simulink model "Arizona_base_GOAT"  (R2022a)
settings: Solver=FixedStepDiscrete  StartTime=0.0  StopTime=inf  FixedStep=Ts  RelTol=1e-3  EnableMultiTasking=on
undefined symbols (not defined in the file): DiscIntNeverNeededParam, Ended, IO307, N_Init, Nref, phi_Init, Single, x_Init, y_Init
libraries: speedgoatlib_fpga_dio x30, speedgoatlib_fpga_quadrature x19, simulink x10, speedgoatlib_IO141 x9, xpcobsoletelib x7, speedgoatlib_fpga x3, cstblocks x3
(part 1 of 3)
settings Model: SimulationMode=external  ExtModeTrigDuration=5  Creator=JBolder  LastModifiedBy=Arizona_PC
settings SolverCC: ConcurrentTasks=on  AlgebraicLoopSolver=TrustRegion  PositivePriorityOrder=on
settings DataIOCC: LimitDataPoints=on  SaveFormat=Array  ReturnWorkspaceOutputs=off  SignalLoggingName=logsOut
settings OptimizationCC: BlockReduction=off  OptimizeBlockIOStorage=off  BufferReuse=off  GlobalBufferReuse=off  ExpressionFolding=off  LocalBlockOutputs=off
settings DebuggingCC: SolverPrmCheckMsg=warning  TasksWithSamePriorityMsg=none  UnconnectedInputMsg=warning  UnconnectedOutputMsg=warning  UnconnectedLineMsg=warning  SFUnexpectedBacktrackingDiag=warning  SFNoUnconditionalDefaultTransitionDiag=warning  SFExecutionAtInitializationDiag=none  SFMachineParentedDataDiag=warning  ArithmeticOperatorsInVariantConditions=warning
settings HardwareCC: ProdBitPerLong=64  ProdLongLongMode=on  ProdHWDeviceType=Intel->x86-64 (Linux 64)
settings ModelReferenceCC: UpdateModelReferenceTargets=Force  EnableParallelModelReferenceBuilds=on  ParallelModelReferenceMATLABWorkerInit=Copy Base Workspace  PropagateVarSize=During execution  PropagateSignalLabelsOutOfModel=off
settings SFSimCC: SimUseLocalCustomCode=off  CustomCodeUndefinedFunction=UseInterfaceOnly  SimTargetLang=C++
settings RTWCC: Description=Simulink Real-Time  SystemTargetFile=slrealtime.tlc  TemplateMakefile=slrealtime_default_tmf  RTWUseLocalCustomCode=off  Toolchain=Simulink Real-Time Toolchain  BuildConfiguration=Faster Runs  CodeExecutionProfiling=on  TargetLang=C++
settings CodeAppCC: StateflowObjectComments=on
settings SimulinkRealTimeTargetCC: UseGCCFastMath=on
settings ConfigComp: CovMetricSettings=dw  CovSaveCumulativeToWorkspaceVar=on  CovSaveSingleToWorkspaceVar=on  CovExternalEMLEnable=off  CovSFcnEnable=off

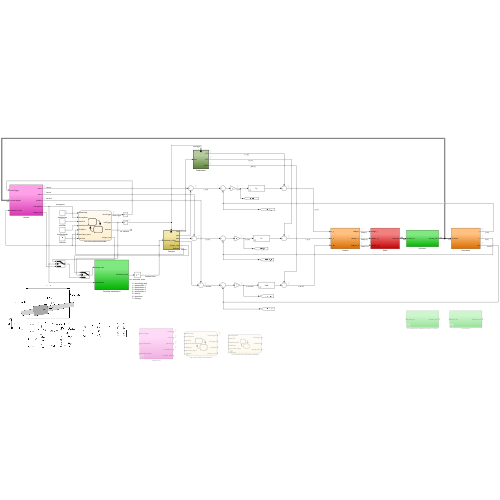
[thumbnail: Simulink's stored preview of the top-level diagram]
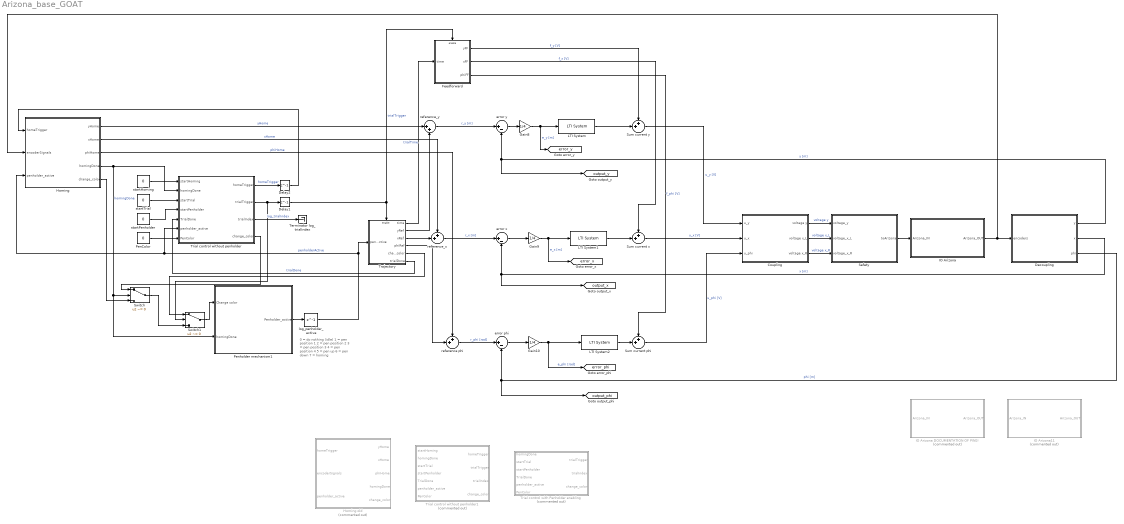
== system Arizona_base_GOAT ==
  note: 0 = do nothing (idle)
      | 1 = pen position 1
      | 2 = pen position 2
      | 3 = pen position 3
      | 4 = pen position 4
      | 5 = pen up
      | 6 = pen down
      | 7 = homing
  Coupling : Subsystem
  Decoupling : Subsystem
  Delay1 : Delay  DelayLength=1  InitialCondition=0
  Delay2 : Delay  DelayLength=1  InitialCondition=0
  Feedforward : Subsystem
  Gain10 : Gain  Gain=1/4
  Gain8 : Gain  Gain=1/4
  Gain9 : Gain  Gain=1/4
  Homing : Subsystem
  Homing old : Subsystem  Commented=on
  IO Arizona : Subsystem
  IO Arizona DOCUMENTATION OF PINS! : Subsystem  Commented=on
  IO Arizona11 : Subsystem  Commented=on
  LTI System : cstblocks/LTI System  sys=Cy  IC=[]
  LTI System1 : cstblocks/LTI System  sys=Cx  IC=[]
  LTI System2 : cstblocks/LTI System  sys=Cphi  IC=[]
  PenColor : Constant  Value=0
  Penholder mechanism1 : Subsystem
  Safety : Subsystem
  Sum current phi : Sum  Inputs=++|
  Sum current x : Sum  Inputs=++|
  Sum current y : Sum  Inputs=++|
  Switch : Switch  Criteria=u2 ~= 0  SaturateOnIntegerOverflow=off  InputSameDT=off
  Switch1 : Switch  Criteria=u2 ~= 0  SaturateOnIntegerOverflow=off  InputSameDT=off
  Terminator log_trialIndex : Terminator
  Trajectory : Subsystem  TreatAsAtomicUnit=on
  Trial control with Penholder enabling : Stateflow chart  Commented=on  TreatAsAtomicUnit=on
  Trial control without penholder : Stateflow chart  TreatAsAtomicUnit=on
  Trial control without penholder1 : Stateflow chart  Commented=on  TreatAsAtomicUnit=on
  error phi : Sum  Inputs=|+-
  error x : Sum  Inputs=|+-
  error y : Sum  Inputs=|+-
  log_penholder_active : Delay  DelayLength=1  InitialCondition=0
  reference phi : Sum  Inputs=++|
  reference_x : Sum  Inputs=++|
  reference_y : Sum  Inputs=|++
  startHoming : Constant  Value=0
  startPenholder : Constant  Value=0
  startTrial : Constant  Value=0
  tag scope: error_phi=global, error_x=global, error_y=global, output_phi=global, output_x=global, output_y=global
  wires:
  Decoupling/2(x) -> [output_x], error x/2  "x [m]"
  IO Arizona/1(Arizona_OUT) -> Homing/2(encoderSignals), Decoupling/1(encoders)
  Safety/1(toArizona) -> IO Arizona/1(Arizona_IN)
  Trajectory/4(phiRef) -> reference phi/2
  startTrial/1 -> Trial control without penholder/3(startTrial)
  Trial control without penholder/3(trialIndex) -> Terminator log_trialIndex/1  "log_trialIndex"
  Delay1/1 -> Trajectory/Enable, Feedforward/Enable  "trialTrigger"
  error y/1 -> Gain8/1
  Homing/4(homingDone) -> Penholder mechanism1/2(homingDone), Switch/2, Trial control without penholder/2(homingDone)  "homingDone"
  reference_y/1 -> error y/1  "r_y [m]"
  Feedforward/1(yFF) -> Sum current y/1  "f_y [V]"
  reference_x/1 -> error x/1  "r_x [m]"
  reference phi/1 -> error phi/1  "r_phi [rad]"
  Sum current y/1 -> Coupling/1(u_y)  "u_y [V]"
  Decoupling/1(y) -> [output_y], error y/2  "y [m]"
  Decoupling/3(phi) -> [output_phi], error phi/2  "phi [m]"
  Sum current x/1 -> Coupling/2(u_x)  "u_x [V]"
  Sum current phi/1 -> Coupling/3(u_phi)  "u_phi [V]"
  log_penholder_active/1 -> Trajectory/1(penholder_active), Homing/3(penholder_active), Trial control without penholder/6(penholder_active)  "penholderActive"
  Trajectory/1(time) -> Feedforward/1(time)  "trialTime"
  Homing/5(change_color) -> Switch/3
  Switch1/1 -> Penholder mechanism1/1(Change color)
  Switch/1 -> Switch1/3
  Trajectory/6(trialDone) -> Trial control without penholder/5(TrialDone)  "trialDone"
  Penholder mechanism1/1(Penholder_active) -> log_penholder_active/1
  Trial control without penholder/4(change_color) -> Switch/1
  Trajectory/5(change_color) -> Switch1/1
  error phi/1 -> Gain10/1
  LTI System2/1 -> Sum current phi/2
  PenColor/1 -> Trial control without penholder/7(PenColor)
  Coupling/2(voltage x_L) -> Safety/2(voltage_x_L)  "voltage x_L"
  Coupling/3(voltage x_R) -> Safety/3(voltage_x_R)  "voltage x_R"
  Trial control without penholder/2(trialTrigger) -> Switch1/2, Delay1/1
  Trial control without penholder/1(homeTrigger) -> Delay2/1  "homeTrigger"
  Delay2/1 -> Homing/1(homeTrigger)
  startHoming/1 -> Trial control without penholder/1(startHoming)
  startPenholder/1 -> Trial control without penholder/4(startPenholder)
  Homing/1(yHome) -> reference_y/1  "yHome"
  Homing/2(xHome) -> reference_x/1  "xHome"
  Homing/3(phiHome) -> reference phi/1  "phiHome"
  Coupling/1(voltage y) -> Safety/1(voltage_y)  "voltage y"
  Gain9/1 -> [error_x], LTI System1/1  "e_x [m]"
  error x/1 -> Gain9/1
  Gain8/1 -> [error_y], LTI System/1  "e_y [m]"
  Gain10/1 -> [error_phi], LTI System2/1  "e_phi [rad]"
  Trajectory/2(yRef) -> reference_y/2
  Feedforward/2(xFF) -> Sum current x/1  "f_x [V]"
  Feedforward/3(phiFF) -> Sum current phi/1  "f_phi [V]"
  Trajectory/3(xRef) -> reference_x/2
  LTI System/1 -> Sum current y/2
  LTI System1/1 -> Sum current x/2

== system Arizona_base_GOAT/Coupling ==
  u_y : Inport
  u_x : Inport  Port=2
  u_phi : Inport  Port=3
  Gain on u_phi : Gain  Gain=1/2.62
  Gain on u_x : Gain  Gain=1/2
  Sum current x_L : Sum  Inputs=|+-
  Sum current x_R : Sum  Inputs=++|
  voltage y : Outport
  voltage x_L : Outport  Port=2
  voltage x_R : Outport  Port=3
  wires:
  u_y/1 -> voltage y/1
  u_x/1 -> Gain on u_x/1
  Gain on u_phi/1 -> Sum current x_L/2, Sum current x_R/2
  Sum current x_L/1 -> voltage x_L/1
  Sum current x_R/1 -> voltage x_R/1
  u_phi/1 -> Gain on u_phi/1
  Gain on u_x/1 -> Sum current x_L/1, Sum current x_R/1

== system Arizona_base_GOAT/Decoupling ==
  encoders : Inport
  Bus Selector : BusSelector  OutputSignals=AI encoders primair.encoder carriage,AI encoders primair.encoder gantry x2,AI encoders primair.encoder gantry x1
  Gain phi : Gain  Gain=1/2.62  OutDataTypeStr=double
  Gain x : Gain  Gain=1/2  OutDataTypeStr=double
  Sum x_L + x_R : Sum  Inputs=|++
  Sum x_R - x_L : Sum  Inputs=-+|
  y : Outport
  x : Outport  Port=2
  phi : Outport  Port=3
  wires:
  encoders/1 -> Bus Selector/1
  Bus Selector/3 -> Sum x_L + x_R/2, Sum x_R - x_L/2  "<encoder gantry x1>"
  Bus Selector/2 -> Sum x_R - x_L/1, Sum x_L + x_R/1  "<encoder gantry x2>"
  Sum x_L + x_R/1 -> Gain x/1
  Sum x_R - x_L/1 -> Gain phi/1
  Gain x/1 -> x/1
  Bus Selector/1 -> y/1  "<encoder carriage>"
  Gain phi/1 -> phi/1

== system Arizona_base_GOAT/Feedforward ==
  time : Inport
  Enable : EnablePort  StatesWhenEnabling=reset
  Direct Lookup Table phiFF : LookupNDDirect  NumberOfTableDimensions=1  TableIsInput=on  Table=[4 5 ;16 19 ]
  Direct Lookup Table xFF : LookupNDDirect  NumberOfTableDimensions=1  TableIsInput=on  Table=[4 5 ;16 19 ]
  Direct Lookup Table yFF : LookupNDDirect  NumberOfTableDimensions=1  TableIsInput=on  Table=[4 5 ;16 19 ]
  set_phiFF : Constant  Value=zeros(Nref,1)
  set_xFF : Constant  Value=zeros(Nref,1)
  set_yFF : Constant  Value=zeros(Nref,1)
  yFF : Outport
  xFF : Outport  Port=2
  phiFF : Outport  Port=3
  wires:
  Direct Lookup Table phiFF/1 -> phiFF/1  "f_phi"
  Direct Lookup Table yFF/1 -> yFF/1  "f_y"
  Direct Lookup Table xFF/1 -> xFF/1  "f_x"
  set_yFF/1 -> Direct Lookup Table yFF/2
  set_xFF/1 -> Direct Lookup Table xFF/2
  time/1 -> Direct Lookup Table yFF/1, Direct Lookup Table xFF/1, Direct Lookup Table phiFF/1
  set_phiFF/1 -> Direct Lookup Table phiFF/2

== system Arizona_base_GOAT/Homing ==
  homeTrigger : Inport
  encoderSignals : Inport  Port=2
  penholder_active : Inport  Port=3
  Enabled subsystem : Subsystem
  Memory block for homing during trials : Subsystem
      settings: PortSchema="{\"entries\":[{\"content\":{\"sides\":[{\"content\":{\"connectorIds\":[\"In1\",\"In2\",\"In3\"]},\"type\":\"ConnectorPlacement.EquallySpacedRectSide\",\"uuid\":\"529cf24d-8a38-49a6-8289-3a46dbfdbf8f\"},{\"content\":{\"connectorIds\":[\"Out1\",\"Out2\",\"Out3\"],\"side\":\"RIGHT\"},\"type\":\"ConnectorPlacement.EquallySpacedRectSide\",\"uuid\":\"39565b64-7967-4644-a7cf-4ede35236997\"},{\"content\":{\"connectorIds\":[\"In4\"],\"side\":\"TOP\"},\"type\":\"ConnectorPlacement.EquallySpacedRectSide\",\"uuid\":\"fd77b9cb-a736-4f15-bdda-ed00ce93e84f\"}]},\"type\":\"ConnectorPlacement.EquallySpacedConnector\",\"uuid\":\"703cf488-7ff6-4b61-bd86-c7430d8b35d0\"}],\"packageUris\":[\"http://schema.mathworks.com/mf0/Connector/R2020b\"],\"version\":\"1.0\"}"
  yHome : Outport
  xHome : Outport  Port=2
  phiHome : Outport  Port=3
  homingDone : Outport  Port=4
  change_color : Outport  Port=5
  tag scope: homingDone=global, phiHome=global, xHome=global, yHome=global
  wires:
  encoderSignals/1 -> Enabled subsystem/1(encoderSignals)
  penholder_active/1 -> Enabled subsystem/2(penholder_active)
  homeTrigger/1 -> Enabled subsystem/Enable, Memory block for homing during trials/4(homeTrigger)
  Enabled subsystem/4(homingDone) -> homingDone/1, [homingDone]
  Memory block for homing during trials/1(yHome_memory) -> yHome/1, [yHome]
  Enabled subsystem/5(change_color) -> change_color/1
  Enabled subsystem/3(phiHome) -> Memory block for homing during trials/3(phiHome)
  Enabled subsystem/2(xHome) -> Memory block for homing during trials/2(xHome)
  Enabled subsystem/1(yHome) -> Memory block for homing during trials/1(yHome)
  Memory block for homing during trials/3(phiHome_memory) -> phiHome/1, [phiHome]
  Memory block for homing during trials/2(xHome_memory) -> xHome/1, [xHome]

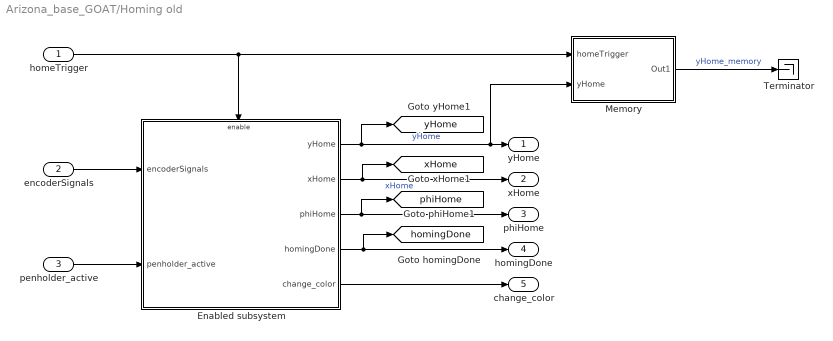
== system Arizona_base_GOAT/Homing old ==
  homeTrigger : Inport
  encoderSignals : Inport  Port=2
  penholder_active : Inport  Port=3
  Enabled subsystem : Subsystem
  Memory : Subsystem
  Terminator : Terminator
  yHome : Outport
  xHome : Outport  Port=2
  phiHome : Outport  Port=3
  homingDone : Outport  Port=4
  change_color : Outport  Port=5
  tag scope: homingDone=global, phiHome=global, xHome=global, yHome=global
  wires:
  encoderSignals/1 -> Enabled subsystem/1(encoderSignals)
  Enabled subsystem/4(homingDone) -> [homingDone], homingDone/1
  Enabled subsystem/2(xHome) -> [xHome], xHome/1  "xHome"
  Enabled subsystem/1(yHome) -> [yHome], Memory/2(yHome), yHome/1  "yHome"
  Enabled subsystem/3(phiHome) -> [phiHome], phiHome/1
  penholder_active/1 -> Enabled subsystem/2(penholder_active)
  Enabled subsystem/5(change_color) -> change_color/1
  homeTrigger/1 -> Enabled subsystem/Enable, Memory/1(homeTrigger)
  Memory/1(Out1) -> Terminator/1  "yHome_memory"

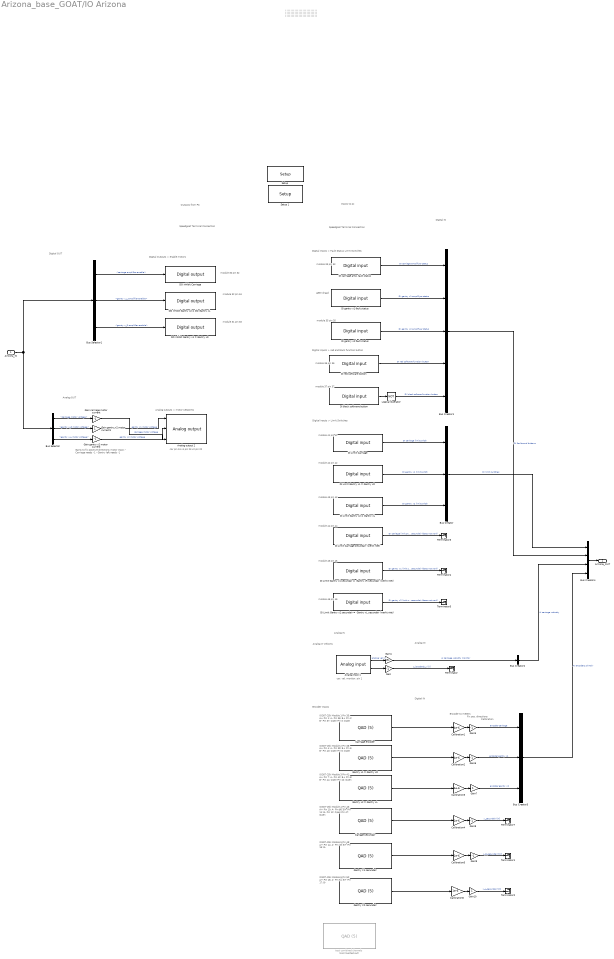
== system Arizona_base_GOAT/IO Arizona ==
  note: Inputs to pc
  note: Digital IN
  note: Speedgoat Terminal Connection
  note: Outputs from PC
  note: Speedgoat Terminal Connection
  note: Digital OUT
  note: |
      | |
      | |
      | |
      | |
      | |
      | |
      | |
      | |
      | |
      | |
      | |
      | |
      | |
      | |
      | |
      | |
      | |
      | |
      | |
      | |
      | |
      | |
      | |
      | |
      | |
      | |
      | |
      | |
      | |
      | |
      | |
      | |
      | |
      | |
      | |
      | |
      | |
      | |
      | |
      | |
      | |
      | |
      | |
      | |
      | |
      | |
      | |
      | |
      | |
      | |
      | |
      | |
      | |
      | |
      | |
      | |
      | |
      | |
      | |
      | |
      | |
      | |
      | |
      | |
      | |
      | |
      | |
      | |
      | |
      | |
      | |
  note: IO307-25k
      | Module 1
      | Pin 35: A+
      | Pin 1: A-
      | Pin 36: B+
      | Pin 2: B-
      | Pin 37: Open
      | Pin 3: Open
  note: Encoder Inputs
  note: IO307-25k
      | Module 4
      | Pin 45: A+
      | Pin 10: A-
      | Pin 46: B+
      | Pin 11: B-
      | Pin 12: Open
      | Pin 47: Open
  note: IO307-25k
      | Module 5
      | Pin 48: A+
      | Pin 14: A-
      | Pin 49: B+
      | Pin 15: B-
  note: IO307-25k
      | Module 2
      | Pin 38: A+
      | Pin 4: A-
      | Pin 39: B+
      | Pin 5: B-
      | Pin 40: Open
      | Pin 6: Open
  note: IO307-25k
      | Module 3
      | Pin 41: A+
      | Pin 7: A-
      | Pin 42: B+
      | Pin 8: B-
      | Pin 44: Open
      | Pin 10: Open
  note: IO307-25k
      | Module 6
      | Pin 50: A+
      | Pin 16: A-
      | Pin 51: B+
      | Pin 17: B-
  note: module 45
      | pin 45
  note: Digital Inputs > Limit Switches
  note: module 41
      | pin 41
  note: module 42
      | pin 42
  note: module 43
      | pin 43
  note: module 44
      | pin 44
  note: module 46
      | pin 46
  note: Digital Outputs > enable motors
  note: module 31
      | pin 33
  note: module 32
      | pin 34
  note: module 30
      | pin 32
  note: Digital inputs > red and black function button
  note: module 35
      | pin 35
  note: Digital Inputs > Fault Status Limit Switches
  note: module 36
      | pin 36
  note: module 37
      | pin 37
  note: module 33
      | pin 33
  note: geen draad
  note: Analog outputs > motor setpoints
  note: car pin 24
      | x1 pin 23
      | x2 pin 22
  note: Analog in Velocity
  note: car. vel. monitor. pin 1
  note: Analog IN
  note: Analog OUT
  note: Gains to fix positive directions motor input:
      | - Carriage needs -1
      | - Gantry left needs -1
  note: Fix pos.
      | directions
  note: Calibration
  note: Analog IN
  note: Encoder
      | to meters
  note: Digital IN
  Arizona_IN : Inport
  Analog input 1 : speedgoatlib_IO141/Analog input   parModuleId=1  parSampleTime=0.001  parPciSlot=-1  parAdcChannels=[4 9]  parAdcNumActiveChannels=[1 1]  parAdcVoltageRange=[5 5 5 5 5 5 5 5 5 5 5 5 5 5 5 5]  parAdcCoupling=[2 2]  parAdcContSampling=0  parAdcDmaEnable=0  parAdcActiveDmaDevices=[1 1 1 1]  parAdcFrameSize=100
      settings: SourceProductName=Simulink Real-Time: Speedgoat I/O Blockset
  Analog output 2 : speedgoatlib_IO141/Analog output   parModuleId=1  parSampleTime=0.001  parPciSlot=-1  parDacChannels=[2 3 4]  parDacVoltageRange=[6 6 6 6]  parDacOverRange=[1 1 1 1]  parDacInitValues=[0 0 0]  parDacReset=[1 1 1]  parDacSyncOut=0  parDacDmaEnable=0  parDacActiveDmaDevices=[1 1 1 1]  parDacDmaLatency=1  parDacFrameSize=100
      settings: SourceProductName=Simulink Real-Time: Speedgoat I/O Blockset
  Bus Creator : BusCreator  Inputs=3
  Bus Creator1 : BusCreator  Inputs=5
  Bus Creator2 : BusCreator  Inputs=1
  Bus Creator3 : BusCreator  Inputs=3
  Bus Creator4 : BusCreator  Inputs=4
  Bus Selector : BusSelector  OutputSignals=carriage motor voltage,gantry x_R motor voltage,gantry x_L motor voltage
  Bus Selector1 : BusSelector  OutputSignals=carriage amplifier enable,gantry x_L amplifier enable,gantry x_R amplifier enable
  Calibration1 : Gain  Gain=4e-6
  Calibration2 : Gain  Gain=4e-6
  Calibration3 : Gain  Gain=4e-6
  Calibration4 : Gain  Gain=1e-6
  Calibration5 : Gain  Gain=1e-6
  Calibration6 : Gain  Gain=1e-6
  Cariage secundair : speedgoatlib_fpga_quadrature/QAD (5)  id=1  chan=4  sampleTime=0.001  enableDma=on  board=IO307-25k  pciSlot=-1  numOfSlots=1  sensorType=Capture A + B Signal  interpolatePosition=on  swapAB=off  indexControlMode=Ignore Index  latchMode=Disabled  gateIndex=No Gating  speedFilterWidth=4  showInputSpeedFilterWidth=off  glitchFilterSeconds=106.7e-9  glitchFilterSecondsEff=108.5e-9  showInputClearPosition=off  showInputClearIndexFound=off  showOutputPosition=off  showOutputTurn=on  showOutputSpeed=off  showOutputIndexFound=off  showOutputLastPulse=off
      settings: SourceProductName=Simulink Real-Time: Speedgoat I/O Blockset
  Carriage encoder : speedgoatlib_fpga_quadrature/QAD (5)  id=1  chan=1  sampleTime=0.001  enableDma=on  board=IO307-25k  pciSlot=-1  numOfSlots=1  sensorType=Capture A + B Signal  interpolatePosition=on  swapAB=off  indexControlMode=Ignore Index  latchMode=Disabled  gateIndex=No Gating  speedFilterWidth=1  showInputSpeedFilterWidth=off  glitchFilterSeconds=106.7e-9  glitchFilterSecondsEff=108.5e-9  showInputClearPosition=off  showInputClearIndexFound=off  showOutputPosition=off  showOutputTurn=on  showOutputSpeed=off  showOutputIndexFound=off  showOutputLastPulse=off
      settings: SourceProductName=Simulink Real-Time: Speedgoat I/O Blockset
  "DI Limit Carriage " : speedgoatlib_fpga_dio/Digital input  id=1  chan=[41]  ts=0.001  pciSlot=-1  board=IO307-25k  vectorizeOutput=off
      settings: SourceProductName=Simulink Real-Time: Speedgoat I/O Blockset
  DI Limit Carriage secundair (werkt niet) : speedgoatlib_fpga_dio/Digital input  id=1  chan=[44]  ts=0.001  pciSlot=-1  board=IO307-25k  vectorizeOutput=off
      settings: SourceProductName=Simulink Real-Time: Speedgoat I/O Blockset
  DI Limit Gantry x1 = Gantry xR : speedgoatlib_fpga_dio/Digital input  id=1  chan=[42]  ts=0.001  pciSlot=-1  board=IO307-25k  vectorizeOutput=off
      settings: SourceProductName=Simulink Real-Time: Speedgoat I/O Blockset
  DI Limit Gantry x1 secundair =  Gantry xR secundair (werkt niet) : speedgoatlib_fpga_dio/Digital input  id=1  chan=[45]  ts=0.001  pciSlot=-1  board=IO307-25k  vectorizeOutput=off
      settings: SourceProductName=Simulink Real-Time: Speedgoat I/O Blockset
  DI Limit Gantry x2 = Gantry xL : speedgoatlib_fpga_dio/Digital input  id=1  chan=[43]  ts=0.001  pciSlot=-1  board=IO307-25k  vectorizeOutput=off
      settings: SourceProductName=Simulink Real-Time: Speedgoat I/O Blockset
  DI Limit Gantry x2 secundair =  Gantry xL secundair (werkt niet) : speedgoatlib_fpga_dio/Digital input  id=1  chan=[46]  ts=0.001  pciSlot=-1  board=IO307-25k  vectorizeOutput=off
      settings: SourceProductName=Simulink Real-Time: Speedgoat I/O Blockset
  DI black software button : speedgoatlib_fpga_dio/Digital input  id=1  chan=[37]  ts=0.001  pciSlot=-1  board=IO307-25k  vectorizeOutput=off
      settings: SourceProductName=Simulink Real-Time: Speedgoat I/O Blockset
  DI carriage amp. fault status : speedgoatlib_fpga_dio/Digital input  id=1  chan=[33]  ts=0.001  pciSlot=-1  board=IO307-25k  vectorizeOutput=off
      settings: SourceProductName=Simulink Real-Time: Speedgoat I/O Blockset
  DI gantry x1 fault status : speedgoatlib_fpga_dio/Digital input  id=1  chan=[34]  ts=0.001  pciSlot=-1  board=IO307-25k  vectorizeOutput=off
      settings: SourceProductName=Simulink Real-Time: Speedgoat I/O Blockset
  DI gantry x2 fault status : speedgoatlib_fpga_dio/Digital input  id=1  chan=[35]  ts=0.001  pciSlot=-1  board=IO307-25k  vectorizeOutput=off
      settings: SourceProductName=Simulink Real-Time: Speedgoat I/O Blockset
  DI red software button : speedgoatlib_fpga_dio/Digital input  id=1  chan=[36]  ts=0.001  pciSlot=-1  board=IO307-25k  vectorizeOutput=off
      settings: SourceProductName=Simulink Real-Time: Speedgoat I/O Blockset
  DO Inhibit Carriage : speedgoatlib_fpga_dio/Digital output  id=1  chan=[30]  init=[0]  reset=[0]  vectorizeInput=off  ts=0.001  pciSlot=-1  board=IO307-25k
      settings: SourceProductName=Simulink Real-Time: Speedgoat I/O Blockset
  DO Inhibit Gantry x1 = Gantry xR : speedgoatlib_fpga_dio/Digital output  id=1  chan=[31]  init=[0]  reset=[0]  vectorizeInput=off  ts=0.001  pciSlot=-1  board=IO307-25k
      settings: SourceProductName=Simulink Real-Time: Speedgoat I/O Blockset
  DO Inhibit Gantry x2 = DO Gantry xL : speedgoatlib_fpga_dio/Digital output  id=1  chan=[32]  init=[0]  reset=[0]  vectorizeInput=off  ts=0.001  pciSlot=-1  board=IO307-25k
      settings: SourceProductName=Simulink Real-Time: Speedgoat I/O Blockset
  Gain{,5..6,8..9} (5 alike) : Gain  Gain=-1
  Gain carriage motor current : Gain  Gain=-1
  Gain gantry x2 motor current : Gain  Gain=-1
  Gain gantry x2 motor current1 : Gain
  Gain1 : Gain  Gain=134
  Gain10 : Gain
  Gain7 : Gain
  Gantry X1 secundair : speedgoatlib_fpga_quadrature/QAD (5)  id=1  chan=5  sampleTime=0.001  enableDma=on  board=IO307-25k  pciSlot=-1  numOfSlots=1  sensorType=Capture A + B Signal  interpolatePosition=on  swapAB=off  indexControlMode=Ignore Index  latchMode=Disabled  gateIndex=No Gating  speedFilterWidth=4  showInputSpeedFilterWidth=off  glitchFilterSeconds=106.7e-9  glitchFilterSecondsEff=108.5e-9  showInputClearPosition=off  showInputClearIndexFound=off  showOutputPosition=off  showOutputTurn=on  showOutputSpeed=off  showOutputIndexFound=off  showOutputLastPulse=off
      settings: SourceProductName=Simulink Real-Time: Speedgoat I/O Blockset
  Gantry x1 = Gantry xR : speedgoatlib_fpga_quadrature/QAD (5)  id=1  chan=2  sampleTime=0.001  enableDma=on  board=IO307-25k  pciSlot=-1  numOfSlots=1  sensorType=Capture A + B Signal  interpolatePosition=on  swapAB=off  indexControlMode=Ignore Index  latchMode=Disabled  gateIndex=No Gating  speedFilterWidth=1  showInputSpeedFilterWidth=off  glitchFilterSeconds=106.7e-9  glitchFilterSecondsEff=108.5e-9  showInputClearPosition=off  showInputClearIndexFound=off  showOutputPosition=off  showOutputTurn=on  showOutputSpeed=off  showOutputIndexFound=off  showOutputLastPulse=off
      settings: SourceProductName=Simulink Real-Time: Speedgoat I/O Blockset
  Gantry x2 = Gantry xL : speedgoatlib_fpga_quadrature/QAD (5)  id=1  chan=3  sampleTime=0.001  enableDma=on  board=IO307-25k  pciSlot=-1  numOfSlots=1  sensorType=Capture A + B Signal  interpolatePosition=on  swapAB=off  indexControlMode=Ignore Index  latchMode=Disabled  gateIndex=No Gating  speedFilterWidth=1  showInputSpeedFilterWidth=off  glitchFilterSeconds=106.7e-9  glitchFilterSecondsEff=108.5e-9  showInputClearPosition=off  showInputClearIndexFound=off  showOutputPosition=off  showOutputTurn=on  showOutputSpeed=off  showOutputIndexFound=off  showOutputLastPulse=off
      settings: SourceProductName=Simulink Real-Time: Speedgoat I/O Blockset
  Gentry X2 secundair : speedgoatlib_fpga_quadrature/QAD (5)  id=1  chan=6  sampleTime=0.001  enableDma=on  board=IO307-25k  pciSlot=-1  numOfSlots=1  sensorType=Capture A + B Signal  interpolatePosition=on  swapAB=off  indexControlMode=Ignore Index  latchMode=Disabled  gateIndex=No Gating  speedFilterWidth=4  showInputSpeedFilterWidth=off  glitchFilterSeconds=106.7e-9  glitchFilterSecondsEff=108.5e-9  showInputClearPosition=off  showInputClearIndexFound=off  showOutputPosition=off  showOutputTurn=on  showOutputSpeed=off  showOutputIndexFound=off  showOutputLastPulse=off
      settings: SourceProductName=Simulink Real-Time: Speedgoat I/O Blockset
  Logical Operator : Logic  Operator=NOT  AllPortsSameDT=off  OutDataTypeStr=boolean
  Setup : speedgoatlib_fpga/Setup/Setup  board=IO307-25k  id=1  device_id=1  frontIO=None  rearIO=None  bitstreamFile=speedgoat_IO307_25k_CI_02479  rev=1.000000  timestamp_string=28/12/21 17:14:03  fpgaFreq=73.73 MHz  fpgaTick=13.56 ns  ProgSpiFlash=off  ProgBPIFlash=off  pciSlot=-1  PullRPort0=pull-up 3.3V  VioPort0=3.3V  PullRPort1=pull-up 3.3V  VioPort1=3.3V  PullRPort2=pull-up 3.3V  VioPort2=3.3V  PullRPort3=pull-up 3.3V  VioPort3=3.3V  PullRPort4=pull-up 3.3V  VioPort4=3.3V  PullRPort5=pull-up 3.3V  VioPort5=3.3V  PullRPort6=pull-up 3.3V  VioPort6=3.3V  PullRPort15=pull-up 3.3V  PullRPort31=pull-up 3.3V  PullRPort47=pull-up 3.3V  PullRPort63=pull-up 3.3V  diffLineTermination_1=on  diffLineTermination_2=on  diffLineTermination_3=on  diffLineTermination_4=on  diffLineTermination_5=on  diffLineTermination_6=on  diffLineTermination_7=on  diffLineTermination_8=on
      settings: SourceProductName=Simulink Real-Time: Speedgoat I/O Blockset
  Setup 1 : speedgoatlib_IO141/Setup   parPciSlot=-1  parModuleId=1  parInterModuleSync=Independent  parConvClockBaseRate=20MHz  parConvClock1Divider=20000  parConvClock2Divider=20000  parFrameTriggerEnable=off  parFrameTriggerDivider=10  parConvClock1BaseRate=1  parConvClock2BaseRate=1  parFrameTriggerClock=1  parAdcCoupling1=Single-Ended  parAdcChannels1=[1 2]  parAdcChannel11=off  parAdcChannel12=off  parAdcChannel13=off  parAdcChannel14=on  parAdcChannel15=off  parAdcChannel16=off  parAdcChannel17=off  parAdcChannel18=off  parAdcRangeAll1=+-10.24 V  parVoltageRangePerChannelEn1=off  parAdcRange11=+-0.64 V  parAdcRange12=+-0.64 V  parAdcRange13=+-0.64 V  parAdcRange14=+-0.64 V  parAdcRange15=+-0.64 V  parAdcRange16=+-0.64 V  parAdcRange17=+-0.64 V  parAdcRange18=+-0.64 V  parAdcCoupling2=Single-Ended  parAdcChannels2=[9 10]  parAdcChannel21=on  parAdcChannel22=off  parAdcChannel23=off  parAdcChannel24=off  parAdcChannel25=off  parAdcChannel26=off  parAdcChannel27=off  parAdcChannel28=off  parAdcRangeAll2=+-10.24 V  parVoltageRangePerChannelEn2=off  parAdcRange21=+-0.64 V  parAdcRange22=+-0.64 V  parAdcRange23=+-0.64 V  parAdcRange24=+-0.64 V  parAdcRange25=+-0.64 V  parAdcRange26=+-0.64 V  parAdcRange27=+-0.64 V  parAdcRange28=+-0.64 V  parAdcChannels=[4 9]  parAdcNumActiveChannels=[1 1]  parAdcVoltageRange=[5 5 5 5 5 5 5 5 5 5 5 5 5 5 5 5]  parAdcCoupling=[2 2]  parAdcContSampling=off  parAdcAutoCorrection=on  parAdcDmaEnable=off  parAdcDmaClock=Clock 1  parAdcFrameSize_=100  parAdcSampleTime_=-1  parAdcActiveDmaDevices=[1 1 1 1]  parAdcFrameTriggerEnable=0  parAdcFrameSize=100  parAdcSampleTime=0.1  parDacChannels=[1 2]  parDacChannel1=off  parDacChannel2=on  parDacChannel3=on  parDacChannel4=on  parDacInitValues=0  parDacResets=1  parDacVoltageRange=[6 6 6 6]  parDacOverRange=[1 1 1 1]  parDacRange1=+-6 V  parDacInitValue1=0  parDacReset1=on  parDacRange2=+-6 V  parDacInitValue2=0  parDacReset2=on  parDacRange3=+-6 V  parDacInitValue3=0  parDacReset3=on  parDacRange4=+-6 V  parDacInitValue4=0  parDacReset4=on  parDacAutoCorrection=on  parDacSyncOut=off  parDacDmaEnable=off  parDacDmaLatency=As small as possible  parDacDmaClock=Clock 1  parDacFrameSize_=100  parDacSampleTime_=-1  parDacActiveDmaDevices=[1 1 1 1]  parDacFrameTriggerEnable=0  parDacFrameSize=100  parDacSampleTime=0.1  parDiChannels=[1 2 3 4 5]  parDoChannels=[6 7 8]  parDioChannel1=In  parDioChannel2=In  parDioChannel3=In  parDioChannel4=In  parDioChannel5=In  parDioChannel6=Out  parDioChannel7=Out  parDioChannel8=Out  parDoInitValues=[0 1 0]  parDoReset=[1 1 1]  parDoInitValue1=0  parDoReset1=on  parDoInitValue2=0  parDoReset2=on  parDoInitValue3=0  parDoReset3=on  parDoInitValue4=0  parDoReset4=on  parDoInitValue5=0  parDoReset5=on  parDoInitValue6=0  parDoReset6=on  parDoInitValue7=1  parDoReset7=on  parDoInitValue8=0  parDoReset8=on  parDiDebounceEnable=off  parDiDebounceTime=0  parDiDebounceValue=0  parDioPullRefFront=Pull-up 3.3 V  parDioPullRefRear=Floating
      settings: SourceProductName=Simulink Real-Time: Speedgoat I/O Blockset
  Terminator{,1..5,7} (7 alike) : Terminator
  test combined channels : speedgoatlib_fpga_quadrature/QAD (5)  Commented=on  id=1  chan=[1:6]  sampleTime=0.001  enableDma=on  board=IO307-25k  pciSlot=-1  numOfSlots=[ones(1,6)]  sensorType=Capture A + B Signal  interpolatePosition=off  swapAB=off  indexControlMode=Ignore Index  latchMode=Disabled  gateIndex=No Gating  speedFilterWidth=4  showInputSpeedFilterWidth=off  glitchFilterSeconds=106.7e-9  glitchFilterSecondsEff=108.5e-9  showInputClearPosition=off  showInputClearIndexFound=off  showOutputPosition=off  showOutputTurn=on  showOutputSpeed=off  showOutputIndexFound=off  showOutputLastPulse=off
      settings: SourceProductName=Simulink Real-Time: Speedgoat I/O Blockset
  Arizona_OUT : Outport
  wires:
  DI black software button/1 -> Logical Operator/1
  Bus Selector1/2 -> DO Inhibit Gantry x2 = DO Gantry xL/1  "<gantry x_L amplifier enable>"
  Gain carriage motor current/1 -> Analog output 2/3  "carriage motor voltage"
  Bus Selector/2 -> Gain gantry x2 motor current1/1  "<gantry x_R motor voltage>"
  Bus Selector1/3 -> DO Inhibit Gantry x1 = Gantry xR/1  "<gantry x_R amplifier enable>"
  Gain gantry x2 motor current1/1 -> Analog output 2/1  "gantry x1 motor voltage"
  Bus Selector/1 -> Gain carriage motor current/1  "<carriage motor voltage>"
  Bus Selector1/1 -> DO Inhibit Carriage/1  "<carriage amplifier enable>"
  Arizona_IN/1 -> Bus Selector1/1, Bus Selector/1
  Gain gantry x2 motor current/1 -> Analog output 2/2  "gantry x2 motor voltage"
  Bus Selector/3 -> Gain gantry x2 motor current/1  "<gantry x_L motor voltage>"
  Gentry X2 secundair/1 -> Calibration6/1
  DI gantry x1 fault status/1 -> Bus Creator1/2  "DI gantry x1 amplifyer status"
  Cariage secundair/1 -> Calibration4/1
  Gain9/1 -> Terminator1/1  "x_R_secundair [m]"
  DI gantry x2 fault status/1 -> Bus Creator1/3  "DI gantry x2 amplifyer status"
  Gain7/1 -> Bus Creator3/3  "encoder gantry x2"
  DI Limit Gantry x2 secundair =  Gantry xL secundair (werkt niet)/1 -> Terminator5/1  "DI gantry x2 limit switch secundair (does not work)"
  Calibration2/1 -> Gain6/1
  Analog input 1/1 -> Gain1/1  "analog vel in"
  Calibration4/1 -> Gain8/1
  Gain5/1 -> Bus Creator3/1  "encoder carriage"
  DI Limit Carriage secundair (werkt niet)/1 -> Terminator3/1  "DI carriage limit switch secundair (does not work)"
  DI Limit Gantry x1 secundair =  Gantry xR secundair (werkt niet)/1 -> Terminator4/1  "DI gantry x1 limit switch secundair (does not work)"
  Gantry X1 secundair/1 -> Calibration5/1
  Gantry x1 = Gantry xR/1 -> Calibration2/1
  Gain6/1 -> Bus Creator3/2  "encoder gantry x1"
  Gantry x2 = Gantry xL/1 -> Calibration3/1
  Carriage encoder/1 -> Calibration1/1
  Bus Creator1/1 -> Bus Creator4/2  "DI faults and buttons"
  Calibration1/1 -> Gain5/1
  Bus Creator4/1 -> Arizona_OUT/1
  DI red software button/1 -> Bus Creator1/4  "DI red software function button"
  Logical Operator/1 -> Bus Creator1/5  "DI black sofware function button"
  Calibration3/1 -> Gain7/1
  Gain1/1 -> Bus Creator2/1  "AI carriage velocity monitor"
  Calibration5/1 -> Gain9/1
  Bus Creator3/1 -> Bus Creator4/4  "AI encoders primair"
  Bus Creator2/1 -> Bus Creator4/3  "AI carriage velocity"
  Gain8/1 -> Terminator7/1  "y_secundair [m]"
  DI Limit Gantry x2 = Gantry xL/1 -> Bus Creator/3  "DI gantry x2 limit switch"
  Gain10/1 -> Terminator2/1  "x_L_secundair [m]"
  DI Limit Gantry x1 = Gantry xR/1 -> Bus Creator/2  "DI gantry x1 limit switch"
  "DI Limit Carriage "/1 -> Bus Creator/1  "DI carriage limit switch"
  DI carriage amp. fault status/1 -> Bus Creator1/1  "DI carriage amplifyer status"
  Bus Creator/1 -> Bus Creator4/1  "DI limit switches"
  Calibration6/1 -> Gain10/1
  Analog input 1/2 -> Gain/1
  Gain/1 -> Terminator/1  "u_loopback_y [V]"

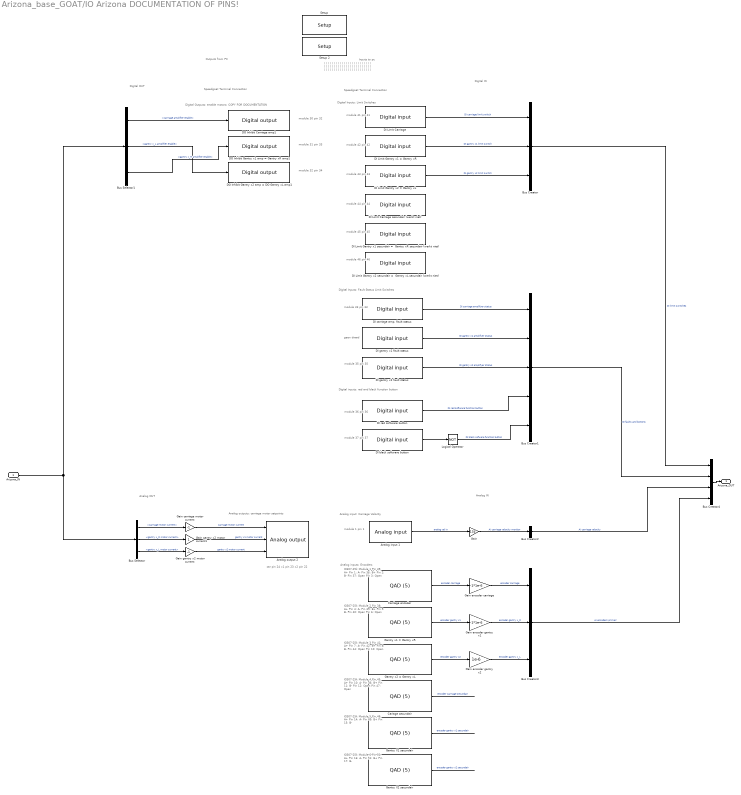
== system Arizona_base_GOAT/IO Arizona DOCUMENTATION OF PINS! ==
  note: Inputs to pc
  note: Analog IN
  note: Digital IN
  note: Speedgoat Terminal Connection
  note: Outputs from PC
  note: Speedgoat Terminal Connection
  note: IO307-25k
      | Module 6
      | Pin 50: A+
      | Pin 16: A-
      | Pin 51: B+
      | Pin 17: B-
  note: IO307-25k
      | Module 1
      | Pin 35: A+
      | Pin 1: A-
      | Pin 36: B+
      | Pin 2: B-
      | Pin 37: Open
      | Pin 3: Open
  note: IO307-25k
      | Module 5
      | Pin 48: A+
      | Pin 14: A-
      | Pin 49: B+
      | Pin 15: B-
  note: IO307-25k
      | Module 2
      | Pin 38: A+
      | Pin 4: A-
      | Pin 39: B+
      | Pin 5: B-
      | Pin 40: Open
      | Pin 6: Open
  note: Analog inputs: Encoders
  note: IO307-25k
      | Module 3
      | Pin 41: A+
      | Pin 7: A-
      | Pin 42: B+
      | Pin 8: B-
      | Pin 44: Open
      | Pin 10: Open
  note: IO307-25k
      | Module 4
      | Pin 45: A+
      | Pin 10: A-
      | Pin 46: B+
      | Pin 11: B-
      | Pin 12: Open
      | Pin 47: Open
  note: Digital Inputs: Limit Switches
  note: module 42
      | pin 42
  note: module 43
      | pin 43
  note: module 41
      | pin 41
  note: module 44
      | pin 44
  note: module 45
      | pin 45
  note: module 46
      | pin 46
  note: Digital Inputs: Fault Status Limit Switches
  note: Digital inputs: red and black function button
  note: module 37
      | pin 37
  note: geen draad
  note: module 33
      | pin 33
  note: module 35
      | pin 35
  note: module 36
      | pin 36
  note: Analog input: Carriage Velocity
  note: module 1
      | pin 1
  note: Digital OUT
  note: Analog OUT
  note: Analog outputs: carriage motor setpoints
  note: car pin 24
      | x1 pin 23
      | x2 pin 22
  note: |
      | |
      | |
      | |
      | |
      | |
      | |
      | |
      | |
      | |
      | |
      | |
      | |
      | |
      | |
      | |
      | |
      | |
      | |
      | |
      | |
      | |
      | |
      | |
      | |
      | |
      | |
      | |
      | |
      | |
      | |
      | |
      | |
      | |
      | |
      | |
      | |
      | |
      | |
      | |
      | |
      | |
      | |
      | |
      | |
      | |
      | |
      | |
      | |
      | |
      | |
      | |
      | |
      | |
      | |
      | |
      | |
      | |
      | |
      | |
      | |
      | |
      | |
      | |
      | |
      | |
      | |
      | |
      | |
      | |
      | |
      | |
  note: Digital Outputs: enable motors: COPY FOR DOCUMENTATION
  note: module 32
      | pin 34
  note: module 31
      | pin 33
  note: module 30
      | pin 32
  Arizona_IN : Inport
  Analog input 1 : speedgoatlib_IO141/Analog input   parModuleId=1  parSampleTime=0.001  parPciSlot=-1  parAdcChannels=4  parAdcNumActiveChannels=[1 0]  parAdcVoltageRange=[5 5 5 5 5 5 5 5 5 5 5 5 5 5 5 5]  parAdcCoupling=[2 1]  parAdcContSampling=0  parAdcDmaEnable=0  parAdcActiveDmaDevices=[1 1 1 1]  parAdcFrameSize=100
      settings: SourceProductName=Simulink Real-Time: Speedgoat I/O Blockset
  Analog output 2 : speedgoatlib_IO141/Analog output   parModuleId=1  parSampleTime=0.001  parPciSlot=-1  parDacChannels=[1 2 3]  parDacVoltageRange=[5 5 5 7]  parDacOverRange=[0 0 0 0]  parDacInitValues=[0 0 0]  parDacReset=[1 1 1]  parDacSyncOut=1  parDacDmaEnable=0  parDacActiveDmaDevices=[1 1 1 1]  parDacDmaLatency=1  parDacFrameSize=100
      settings: SourceProductName=Simulink Real-Time: Speedgoat I/O Blockset
  Bus Creator : BusCreator  Inputs=3
  Bus Creator1 : BusCreator  Inputs=5
  Bus Creator2 : BusCreator  Inputs=1
  Bus Creator3 : BusCreator  Inputs=3
  Bus Creator4 : BusCreator  Inputs=4
  Bus Selector : BusSelector  OutputSignals=carriage motor current,gantry x_R motor current,gantry x_L motor current
  Bus Selector1 : BusSelector  OutputSignals=carriage amplifier enable,gantry x_L amplifier enable,gantry x_R amplifier enable
  Cariage secundair : speedgoatlib_fpga_quadrature/QAD (5)  id=1  chan=[4]  sampleTime=0.001  enableDma=on  board=IO307-25k  pciSlot=-1  numOfSlots=[1]  sensorType=Capture A + B Signal  interpolatePosition=off  swapAB=off  indexControlMode=Ignore Index  latchMode=Disabled  gateIndex=No Gating  speedFilterWidth=4  showInputSpeedFilterWidth=off  glitchFilterSeconds=106.7e-9  glitchFilterSecondsEff=108.5e-9  showInputClearPosition=off  showInputClearIndexFound=off  showOutputPosition=off  showOutputTurn=on  showOutputSpeed=off  showOutputIndexFound=off  showOutputLastPulse=off
      settings: SourceProductName=Simulink Real-Time: Speedgoat I/O Blockset
  Carriage encoder : speedgoatlib_fpga_quadrature/QAD (5)  id=1  chan=[1]  sampleTime=0.001  enableDma=on  board=IO307-25k  pciSlot=-1  numOfSlots=[1]  sensorType=Capture A + B Signal  interpolatePosition=off  swapAB=off  indexControlMode=Ignore Index  latchMode=Disabled  gateIndex=No Gating  speedFilterWidth=4  showInputSpeedFilterWidth=off  glitchFilterSeconds=106.7e-9  glitchFilterSecondsEff=108.5e-9  showInputClearPosition=off  showInputClearIndexFound=off  showOutputPosition=off  showOutputTurn=on  showOutputSpeed=off  showOutputIndexFound=off  showOutputLastPulse=off
      settings: SourceProductName=Simulink Real-Time: Speedgoat I/O Blockset
  "DI Limit Carriage " : speedgoatlib_fpga_dio/Digital input  id=1  chan=[41]  ts=0.001  pciSlot=-1  board=IO307-25k  vectorizeOutput=off
      settings: SourceProductName=Simulink Real-Time: Speedgoat I/O Blockset
  DI Limit Carriage secundair (werkt niet) : speedgoatlib_fpga_dio/Digital input  id=1  chan=[44]  ts=0.001  pciSlot=-1  board=IO307-25k  vectorizeOutput=off
      settings: SourceProductName=Simulink Real-Time: Speedgoat I/O Blockset
  DI Limit Gantry x1 = Gantry xR : speedgoatlib_fpga_dio/Digital input  id=1  chan=[42]  ts=0.001  pciSlot=-1  board=IO307-25k  vectorizeOutput=off
      settings: SourceProductName=Simulink Real-Time: Speedgoat I/O Blockset
  DI Limit Gantry x1 secundair =  Gantry xR secundair (werkt niet) : speedgoatlib_fpga_dio/Digital input  id=1  chan=[45]  ts=0.001  pciSlot=-1  board=IO307-25k  vectorizeOutput=off
      settings: SourceProductName=Simulink Real-Time: Speedgoat I/O Blockset
  DI Limit Gantry x2 = Gantry xL : speedgoatlib_fpga_dio/Digital input  id=1  chan=[43]  ts=0.001  pciSlot=-1  board=IO307-25k  vectorizeOutput=off
      settings: SourceProductName=Simulink Real-Time: Speedgoat I/O Blockset
  DI Limit Gantry x2 secundair =  Gantry xL secundair (werkt niet) : speedgoatlib_fpga_dio/Digital input  id=1  chan=[46]  ts=0.001  pciSlot=-1  board=IO307-25k  vectorizeOutput=off
      settings: SourceProductName=Simulink Real-Time: Speedgoat I/O Blockset
  DI black software button : speedgoatlib_fpga_dio/Digital input  id=1  chan=[37]  ts=0.001  pciSlot=-1  board=IO307-25k  vectorizeOutput=off
      settings: SourceProductName=Simulink Real-Time: Speedgoat I/O Blockset
  DI carriage amp. fault status : speedgoatlib_fpga_dio/Digital input  id=1  chan=[33]  ts=0.001  pciSlot=-1  board=IO307-25k  vectorizeOutput=off
      settings: SourceProductName=Simulink Real-Time: Speedgoat I/O Blockset
  DI gantry x1 fault status : speedgoatlib_fpga_dio/Digital input  id=1  chan=[34]  ts=0.001  pciSlot=-1  board=IO307-25k  vectorizeOutput=off
      settings: SourceProductName=Simulink Real-Time: Speedgoat I/O Blockset
  DI gantry x2 fault status : speedgoatlib_fpga_dio/Digital input  id=1  chan=[35]  ts=0.001  pciSlot=-1  board=IO307-25k  vectorizeOutput=off
      settings: SourceProductName=Simulink Real-Time: Speedgoat I/O Blockset
  DI red software button : speedgoatlib_fpga_dio/Digital input  id=1  chan=[36]  ts=0.001  pciSlot=-1  board=IO307-25k  vectorizeOutput=off
      settings: SourceProductName=Simulink Real-Time: Speedgoat I/O Blockset
  DO Inhibit Carriage amp1 : speedgoatlib_fpga_dio/Digital output  id=1  chan=[30]  init=[0]  reset=[0]  vectorizeInput=off  ts=0.001  pciSlot=-1  board=IO307-25k
      settings: SourceProductName=Simulink Real-Time: Speedgoat I/O Blockset
  DO Inhibit Gantry x1 amp = Gantry xR amp1 : speedgoatlib_fpga_dio/Digital output  id=1  chan=[31]  init=[0]  reset=[0]  vectorizeInput=off  ts=0.001  pciSlot=-1  board=IO307-25k
      settings: SourceProductName=Simulink Real-Time: Speedgoat I/O Blockset
  DO Inhibit Gantry x2 amp = DO Gantry xL amp1 : speedgoatlib_fpga_dio/Digital output  id=1  chan=[32]  init=[0]  reset=[0]  vectorizeInput=off  ts=0.001  pciSlot=-1  board=IO307-25k
      settings: SourceProductName=Simulink Real-Time: Speedgoat I/O Blockset
  Gain : Gain  Gain=134
  Gain carriage motor current : Gain  Gain=-1
  Gain encoder carriage : Gain  Gain=-1*1e-6
  Gain encoder gantry x1 : Gain  Gain=-1*1e-6
  Gain encoder gantry x2 : Gain  Gain=1e-6
  Gain gantry x2 motor current : Gain  Gain=-1
  Gain gantry x2 motor current1 : Gain
  Gantry X1 secundair : speedgoatlib_fpga_quadrature/QAD (5)  id=1  chan=[5]  sampleTime=0.001  enableDma=on  board=IO307-25k  pciSlot=-1  numOfSlots=[1]  sensorType=Capture A + B Signal  interpolatePosition=off  swapAB=off  indexControlMode=Ignore Index  latchMode=Disabled  gateIndex=No Gating  speedFilterWidth=4  showInputSpeedFilterWidth=off  glitchFilterSeconds=106.7e-9  glitchFilterSecondsEff=108.5e-9  showInputClearPosition=off  showInputClearIndexFound=off  showOutputPosition=off  showOutputTurn=on  showOutputSpeed=off  showOutputIndexFound=off  showOutputLastPulse=off
      settings: SourceProductName=Simulink Real-Time: Speedgoat I/O Blockset
  Gantry x1 = Gantry xR : speedgoatlib_fpga_quadrature/QAD (5)  id=1  chan=[2]  sampleTime=0.001  enableDma=on  board=IO307-25k  pciSlot=-1  numOfSlots=[1]  sensorType=Capture A + B Signal  interpolatePosition=off  swapAB=off  indexControlMode=Ignore Index  latchMode=Disabled  gateIndex=No Gating  speedFilterWidth=4  showInputSpeedFilterWidth=off  glitchFilterSeconds=106.7e-9  glitchFilterSecondsEff=108.5e-9  showInputClearPosition=off  showInputClearIndexFound=off  showOutputPosition=off  showOutputTurn=on  showOutputSpeed=off  showOutputIndexFound=off  showOutputLastPulse=off
      settings: SourceProductName=Simulink Real-Time: Speedgoat I/O Blockset
  Gantry x2 = Gantry xL : speedgoatlib_fpga_quadrature/QAD (5)  id=1  chan=[3]  sampleTime=0.001  enableDma=on  board=IO307-25k  pciSlot=-1  numOfSlots=[1]  sensorType=Capture A + B Signal  interpolatePosition=off  swapAB=off  indexControlMode=Ignore Index  latchMode=Disabled  gateIndex=No Gating  speedFilterWidth=4  showInputSpeedFilterWidth=off  glitchFilterSeconds=106.7e-9  glitchFilterSecondsEff=108.5e-9  showInputClearPosition=off  showInputClearIndexFound=off  showOutputPosition=off  showOutputTurn=on  showOutputSpeed=off  showOutputIndexFound=off  showOutputLastPulse=off
      settings: SourceProductName=Simulink Real-Time: Speedgoat I/O Blockset
  Gentry X2 secundair : speedgoatlib_fpga_quadrature/QAD (5)  id=1  chan=[6]  sampleTime=0.001  enableDma=on  board=IO307-25k  pciSlot=-1  numOfSlots=[1]  sensorType=Capture A + B Signal  interpolatePosition=off  swapAB=off  indexControlMode=Ignore Index  latchMode=Disabled  gateIndex=No Gating  speedFilterWidth=4  showInputSpeedFilterWidth=off  glitchFilterSeconds=106.7e-9  glitchFilterSecondsEff=108.5e-9  showInputClearPosition=off  showInputClearIndexFound=off  showOutputPosition=off  showOutputTurn=on  showOutputSpeed=off  showOutputIndexFound=off  showOutputLastPulse=off
      settings: SourceProductName=Simulink Real-Time: Speedgoat I/O Blockset
  Logical Operator : Logic  Operator=NOT  AllPortsSameDT=off  OutDataTypeStr=boolean
  Setup : speedgoatlib_fpga/Setup/Setup  board=IO307-25k  id=1  device_id=1  frontIO=None  rearIO=None  bitstreamFile=speedgoat_IO307_25k_CI_02479  rev=1.000000  timestamp_string=28/12/21 17:14:03  fpgaFreq=73.73 MHz  fpgaTick=13.56 ns  ProgSpiFlash=off  ProgBPIFlash=off  pciSlot=-1  PullRPort0=pull-up 3.3V  VioPort0=3.3V  PullRPort1=pull-up 3.3V  VioPort1=3.3V  PullRPort2=pull-up 3.3V  VioPort2=3.3V  PullRPort3=pull-up 3.3V  VioPort3=3.3V  PullRPort4=pull-up 3.3V  VioPort4=3.3V  PullRPort5=pull-up 3.3V  VioPort5=3.3V  PullRPort6=pull-up 3.3V  VioPort6=3.3V  PullRPort15=pull-up 3.3V  PullRPort31=pull-up 3.3V  PullRPort47=pull-up 3.3V  PullRPort63=pull-up 3.3V  diffLineTermination_1=on  diffLineTermination_2=on  diffLineTermination_3=on  diffLineTermination_4=on  diffLineTermination_5=on  diffLineTermination_6=on  diffLineTermination_7=on  diffLineTermination_8=on
      settings: SourceProductName=Simulink Real-Time: Speedgoat I/O Blockset
  Setup 2 : speedgoatlib_IO141/Setup   parPciSlot=-1  parModuleId=1  parInterModuleSync=Independent  parConvClockBaseRate=20MHz  parConvClock1Divider=20000  parConvClock2Divider=20000  parFrameTriggerEnable=off  parFrameTriggerDivider=10  parConvClock1BaseRate=1  parConvClock2BaseRate=1  parFrameTriggerClock=1  parAdcCoupling1=Single-Ended  parAdcChannels1=[1 2]  parAdcChannel11=off  parAdcChannel12=off  parAdcChannel13=off  parAdcChannel14=on  parAdcChannel15=off  parAdcChannel16=off  parAdcChannel17=off  parAdcChannel18=off  parAdcRangeAll1=+-10.24 V  parVoltageRangePerChannelEn1=off  parAdcRange11=+-0.64 V  parAdcRange12=+-0.64 V  parAdcRange13=+-0.64 V  parAdcRange14=+-0.64 V  parAdcRange15=+-0.64 V  parAdcRange16=+-0.64 V  parAdcRange17=+-0.64 V  parAdcRange18=+-0.64 V  parAdcCoupling2=Differential  parAdcChannels2=[9 10]  parAdcChannel21=off  parAdcChannel22=off  parAdcChannel23=off  parAdcChannel24=off  parAdcChannel25=off  parAdcChannel26=off  parAdcChannel27=off  parAdcChannel28=off  parAdcRangeAll2=+-10.24 V  parVoltageRangePerChannelEn2=off  parAdcRange21=+-0.64 V  parAdcRange22=+-0.64 V  parAdcRange23=+-0.64 V  parAdcRange24=+-0.64 V  parAdcRange25=+-0.64 V  parAdcRange26=+-0.64 V  parAdcRange27=+-0.64 V  parAdcRange28=+-0.64 V  parAdcChannels=4  parAdcNumActiveChannels=[1 0]  parAdcVoltageRange=[5 5 5 5 5 5 5 5 5 5 5 5 5 5 5 5]  parAdcCoupling=[2 1]  parAdcContSampling=off  parAdcAutoCorrection=on  parAdcDmaEnable=off  parAdcDmaClock=Clock 1  parAdcFrameSize_=100  parAdcSampleTime_=-1  parAdcActiveDmaDevices=[1 1 1 1]  parAdcFrameTriggerEnable=0  parAdcFrameSize=100  parAdcSampleTime=0.1  parDacChannels=[1 2]  parDacChannel1=on  parDacChannel2=on  parDacChannel3=on  parDacChannel4=off  parDacInitValues=0  parDacResets=1  parDacVoltageRange=[5 5 5 7]  parDacOverRange=[0 0 0 0]  parDacRange1=+-5 V  parDacInitValue1=0  parDacReset1=on  parDacRange2=+-5 V  parDacInitValue2=0  parDacReset2=on  parDacRange3=+-5 V  parDacInitValue3=0  parDacReset3=on  parDacRange4=+-10 V  parDacInitValue4=0  parDacReset4=on  parDacAutoCorrection=on  parDacSyncOut=on  parDacDmaEnable=off  parDacDmaLatency=As small as possible  parDacDmaClock=Clock 1  parDacFrameSize_=100  parDacSampleTime_=-1  parDacActiveDmaDevices=[1 1 1 1]  parDacFrameTriggerEnable=0  parDacFrameSize=100  parDacSampleTime=0.1  parDiChannels=[1 2 3 4 5]  parDoChannels=[6 7 8]  parDioChannel1=In  parDioChannel2=In  parDioChannel3=In  parDioChannel4=In  parDioChannel5=In  parDioChannel6=Out  parDioChannel7=Out  parDioChannel8=Out  parDoInitValues=[0 0 0]  parDoReset=[1 1 1]  parDoInitValue1=0  parDoReset1=on  parDoInitValue2=0  parDoReset2=on  parDoInitValue3=0  parDoReset3=on  parDoInitValue4=0  parDoReset4=on  parDoInitValue5=0  parDoReset5=on  parDoInitValue6=0  parDoReset6=on  parDoInitValue7=0  parDoReset7=on  parDoInitValue8=0  parDoReset8=on  parDiDebounceEnable=off  parDiDebounceTime=0  parDiDebounceValue=0  parDioPullRefFront=Pull-up 3.3 V  parDioPullRefRear=Floating
      settings: SourceProductName=Simulink Real-Time: Speedgoat I/O Blockset
  Arizona_OUT : Outport
  wires:
  DI Limit Gantry x2 = Gantry xL/1 -> Bus Creator/3  "DI gantry x2 limit switch"
  Arizona_IN/1 -> Bus Selector1/1, Bus Selector/1
  Bus Creator3/1 -> Bus Creator4/4  "AI encoders primair"
  Bus Creator2/1 -> Bus Creator4/3  "AI carriage velocity"
  Bus Creator1/1 -> Bus Creator4/2  "DI faults and buttons"
  Bus Creator/1 -> Bus Creator4/1  "DI limit switches"
  Gain carriage motor current/1 -> Analog output 2/1  "carriage motor current"
  Bus Selector/3 -> Gain gantry x2 motor current/1  "<gantry x_L motor current>"
  Bus Selector1/3 -> DO Inhibit Gantry x1 amp = Gantry xR amp1/1  "<gantry x_R amplifier enable>"
  DI black software button/1 -> Logical Operator/1
  Logical Operator/1 -> Bus Creator1/5  "DI black sofware function button"
  DI gantry x1 fault status/1 -> Bus Creator1/2  "DI gantry x1 amplifyer status"
  DI gantry x2 fault status/1 -> Bus Creator1/3  "DI gantry x2 amplifyer status"
  Bus Selector/2 -> Gain gantry x2 motor current1/1  "<gantry x_R motor current>"
  Gain encoder carriage/1 -> Bus Creator3/1  "encoder carriage"
  Bus Selector1/2 -> DO Inhibit Gantry x2 amp = DO Gantry xL amp1/1  "<gantry x_L amplifier enable>"
  Bus Selector1/1 -> DO Inhibit Carriage amp1/1  "<carriage amplifier enable>"
  Gantry x1 = Gantry xR/1 -> Gain encoder gantry x1/1  "encoder gantry x1"
  DI red software button/1 -> Bus Creator1/4  "DI red software function button"
  DI Limit Gantry x1 = Gantry xR/1 -> Bus Creator/2  "DI gantry x1 limit switch"
  Gain encoder gantry x1/1 -> Bus Creator3/2  "encoder gantry x_R"
  DI carriage amp. fault status/1 -> Bus Creator1/1  "DI carriage amplifyer status"
  "DI Limit Carriage "/1 -> Bus Creator/1  "DI carriage limit switch"
  Carriage encoder/1 -> Gain encoder carriage/1  "encoder carriage"
  Bus Selector/1 -> Gain carriage motor current/1  "<carriage motor current>"
  Gantry x2 = Gantry xL/1 -> Gain encoder gantry x2/1  "encoder gantry x2"
  Gain gantry x2 motor current/1 -> Analog output 2/3  "gantry x2 motor current"
  Gain encoder gantry x2/1 -> Bus Creator3/3  "encoder gantry x_L"
  Gain/1 -> Bus Creator2/1  "AI carriage velocity monitor"
  Bus Creator4/1 -> Arizona_OUT/1
  Gain gantry x2 motor current1/1 -> Analog output 2/2  "gantry x1 motor current"
  Analog input 1/1 -> Gain/1  "analog vel in"
  Gentry X2 secundair/1 -> ?  "encoder gantry x2 secundair"
  Gantry X1 secundair/1 -> ?  "encoder gantry x1 secundair"
  Cariage secundair/1 -> ?  "encoder carriage secundair"
